simulink library "sm_rollerV_lib_lower_frame_idlerArm_i2u0l3"  (R2026a)
settings: Solver=VariableStepAuto
undefined symbols (not defined in the file): Fixed, Right, Trac
libraries: sm_rollerV_lib_underc_elem x1, sm_rollerV_lib_underc_idlerArm_i2u0l3 x1
Description:
  | Copyright 2024-2026 The MathWorks, Inc.
settings Model: Creator=smiller  LastModifiedBy=smiller

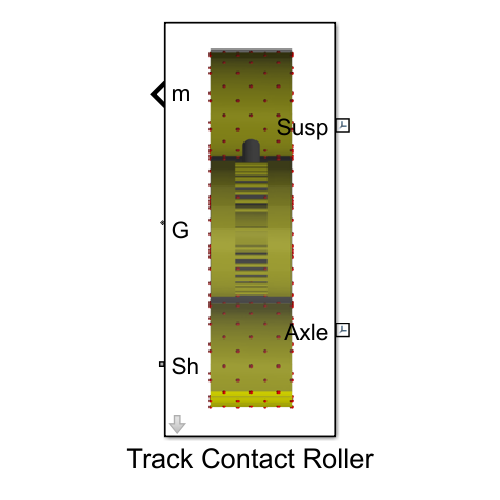
[thumbnail: Simulink's stored preview of the top-level diagram]
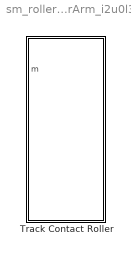
== system sm_rollerV_lib_lower_frame_idlerArm_i2u0l3 ==
  Track Contact Roller : Subsystem  mask(Lower Frame with Roller Point Cloud Contact Geometry){sprk_wid_roll=Trac.Sprocket.Roller.wid, sprk_rad_roll=Trac.Sprocket.Roller.rad, sprk_clr=Trac.Sprocket.Roller.clr, sprk_opc=Trac.Sprocket.Roller.opc, sprk_rad_pitch=Trac.Sprocket.Spoke.pitch_rad, sprk_spoke_rad=Trac.Sprocket.Spoke.rad, sprk_spoke_num=Trac.Sprocket.nSpokes, sprk_spoke_len=Trac.Sprocket.Spoke.len, sprk_rim_spoke_xc=Trac.Sprocket.Rim.spoke_xc, sprk_rim_ir=Trac.Sprocket.Rim.rad_inner, sprk_rim_thk=Trac.Sprocket.Rim.thk, idlerR_rad=Trac.IdlerR.rad, idlerF_rad=Trac.IdlerF.rad, idlerR_total_len=Trac.IdlerR.len_total, idlerF_total_len=Trac.IdlerF.len_total, idlerR_avg_rho=Trac.IdlerR.rho_avg, idlerF_avg_rho=Trac.IdlerF.rho_avg, idlerR_clr=Trac.IdlerR.clr, idlerF_clr=Trac.IdlerF.clr, idlerR_opc=Trac.IdlerR.opc, idlerF_opc=Trac.IdlerF.opc, idlerR_contgeo_ptcld=Trac.IdlerR.ground_contact.ptcld.pts, idlerF_contgeo_ptcld=Trac.IdlerF.ground_contact.ptcld.pts, idlerR_contgeo_rad=Trac.IdlerR.ground_contact.ptcld.rad, idlerF_contgeo_rad=Trac.IdlerF.ground_contact.ptcld.rad, idlerR_contgeo_clr=Trac.IdlerR.belt_contact.clr, idlerF_contgeo_clr=Trac.IdlerF.belt_contact.clr, idlerR_contgeo_opc=Trac.IdlerR.belt_contact.opc, idlerF_contgeo_opc=Trac.IdlerF.belt_contact.opc, arm_idlerc=Trac.IdlerArm.Pivot_to_Idler, arm_tens_x=Trac.IdlerArm.Pivot_to_TensionerX, arm_tens_y=Trac.IdlerArm.Pivot_to_TensionerY, arm_wid=Trac.IdlerArm.wid, arm_thk=Trac.IdlerArm.thk, arm_rho=Trac.IdlerArm.rho, arm_clr=Trac.IdlerArm.clr, arm_opc=Trac.IdlerArm.opc, roller_lower_rad=Trac.Roller.Lower.rad, roller_lower_len=Trac.Roller.Lower.len, roller_lower_rho=Trac.Roller.Lower.rho, roller_lower_clr=Trac.Roller.Lower.clr, roller_lower_opc=Trac.Roller.Lower.opc, roller_lower_contgeo_ptcld=Trac.Roller.Lower.ground_contact.ptcld.pts, roller_lower_contgeo_rad=Trac.Roller.Lower.ground_contact.ptcld.rad, roller_lower_contgeo_clr=Trac.Roller.Lower.belt_contact.clr, roller_lower_contgeo_opc=Trac.Roller.Lower.belt_contact.opc, tensioner_cyl_len=Trac.IdlerF.Tensioner.cyl.len, tensioner_cyl_rad=Trac.IdlerF.Tensioner.cyl.rad, tensioner_cyl_rho=Trac.IdlerF.Tensioner.cyl.rho, tensioner_cyl_clr=Trac.IdlerF.Tensioner.cyl.clr, tensioner_cyl_opc=Trac.IdlerF.Tensioner.cyl.opc, tensioner_pist_len=Trac.IdlerF.Tensioner.piston.len, tensioner_pist_rad=Trac.IdlerF.Tensioner.piston.rad, tensioner_pist_rho=Trac.IdlerF.Tensioner.piston.rho, tensioner_pist_clr=Trac.IdlerF.Tensioner.piston.clr, tensioner_pist_opc=Trac.IdlerF.Tensioner.piston.opc, tensioner_br_len=Trac.IdlerF.Tensioner.bracket.len, tensioner_br_width=Trac.IdlerF.Tensioner.bracket.wid, tensioner_br_height=Trac.IdlerF.Tensioner.bracket.height, tensioner_br_thk=Trac.IdlerF.Tensioner.bracket.thk, tensioner_br_rho=Trac.IdlerF.Tensioner.bracket.rho, tensioner_br_clr=Trac.IdlerF.Tensioner.bracket.clr, tensioner_br_opc=Trac.IdlerF.Tensioner.bracket.opc, tensioner_eqpos=Trac.IdlerF.Tensioner.xeq, tensioner_x0=Trac.IdlerF.Tensioner.x0, tensioner_k=Trac.IdlerF.Tensioner.K, tensioner_b=Trac.IdlerF.Tensioner.B, popup_leftOrRight=Right, popup_trackFrame=Fixed, roller_lower_x=Trac.Frame.SprkOffLon.Lower, idlerFix_x=Trac.Frame.SprkOffLon.IdlerR, idlerArm_x=Trac.Frame.SprkOffLon.IdlerArm, tensionC_x=Trac.Frame.SprkOffLon.TensionC, frame_pivot_x=Trac.Frame.SprkOffLon.PivotFra, axle_x=Trac.Frame.SprkOffLon.Axle, roller_lower_y=Trac.Frame.SprkOffVer.Lower, idlerFix_y=Trac.Frame.SprkOffVer.IdlerR, tensionC_y=Trac.Frame.SprkOffVer.TensionC, frame_pivot_y=Trac.Frame.SprkOffVer.PivotFra, axle_y=Trac.Frame.SprkOffVer.Axle, idlerArm_y=Trac.Frame.SprkOffVer.IdlerArm, frame_mass=Trac.Frame.TrackFrame.Mass, frame_cg_offset=Trac.Frame.TrackFrame.CG, frame_moi=Trac.Frame.TrackFrame.MOI, frame_poi=Trac.Frame.TrackFrame.POI, frame_roller_cg_offset=Trac.Frame.SprkFrame.CG, frame_roller_mass=Trac.Frame.SprkFrame.Mass, frame_roller_moi=Trac.Frame.SprkFrame.MOI, frame_roller_poi=Trac.Frame.SprkFrame.POI, frame_susp_offset=Trac.Frame.SuspOffset, roller_frame_pivot_range=Trac.Frame.PivotFra.Range, roller_frame_pivot_k=Trac.Frame.PivotFra.LimitK, roller_frame_pivot_b=Trac.Frame.PivotFra.LimitB, roller_frame_pivot_tw=Trac.Frame.PivotFra.LimitTW, sprk_rolling_rad=Trac.Sprocket.ground_contact.rolling_radius, roller_lower_rolling_rad=Trac.Roller.Lower.ground_contact.rolling_radius, idlerF_rolling_rad=Trac.IdlerF.ground_contact.rolling_radius, idlerR_rolling_rad=Trac.IdlerR.ground_contact.rolling_radius, rolling_cyl_len=Trac.Belt.w, accent_vis_lext=1e-3, roller_lower_cyl_clr=Trac.Roller.Lower.clr, roller_lower_cyl_opc=Trac.Roller.Lower.opc, idlerR_rollvervis_clr=Trac.IdlerR.clr, idlerF_rollvervis_clr=Trac.IdlerF.clr, idlerR_rollervis_opc=Trac.IdlerR.opc, idlerF_rollervis_opc=Trac.IdlerF.opc, accMn=0.65, accMx=0.75, acc_clr=[0.8 0.8 0.8], acc_opc=1, track_m=Trac.Vis.Track.m, track_cg_offset=Trac.Vis.Track.cg, track_moi=Trac.Vis.Track.moi, track_poi=Trac.Vis.Track.poi, track_xc=Trac.Vis.Track.track_xc, track_clr=Trac.Vis.Track.clr, track_opc=Trac.Vis.Track.opc, popup_sense_roller=Actuator Torque}
      mask prompts: sprk_wid_roll "Roller Width (m)"; sprk_rad_roll "Rolling Radius (m)"; sprk_clr "Color [R G B] (0-1)"; sprk_opc "Opacity (0-1)"; sprk_rad_pitch "Pitch Radius (m)"; sprk_spoke_rad "Radius (m)"; sprk_spoke_num "Number of Spokes"; sprk_spoke_len "Length (m)"; sprk_rim_spoke_xc "Spoke Cross Section [x y] (m)"; sprk_rim_ir "Inner Radius (m)"; sprk_rim_thk "Thickness (m)"; arm_idlerc "Offset Pivot to Idler Center (m)"; arm_tens_x "Offset Pivot to Tensioner Long. (m)"; arm_tens_y "Offset Pivot to Tensioner Vert. (m)"; arm_wid "Idler Arm Width (m)"; arm_thk "Idler Arm Thickness (m)"; arm_rho "Idler Arm Density"; arm_clr "Idler Arm Color [R G B] (m) (0-1)"; arm_opc "Opacity (0-1)"; roller_lower_rad "Radius (m)"; roller_lower_len "Length (m)"; roller_lower_rho "Density (kg/m^3)"; roller_lower_clr "Color [R G B] (0-1)"; roller_lower_opc "Opacity (0-1)"; roller_lower_contgeo_ptcld "Point Cloud [x y z] (m)"; roller_lower_contgeo_rad "Radius (m)"; roller_lower_contgeo_clr "Color [R G B] (0-1)"; roller_lower_contgeo_opc "Opacity (0-1)"; tensioner_cyl_len "Length (m)"; tensioner_cyl_rad "Radius (m)"; tensioner_cyl_rho "Density (kg/m^3)"; tensioner_cyl_clr "Color [R G B] (0-1)"; tensioner_cyl_opc "Opacity (0-1)"; tensioner_pist_len "Piston Length (m)"; tensioner_pist_rad "Radius (m)"; tensioner_pist_rho "Density (kg/m^3)"; tensioner_pist_clr "Color [R G B] (0-1)"; tensioner_pist_opc "Opacity (0.1)"; tensioner_br_len "Length (m)"; tensioner_br_width "Width (m)"; tensioner_br_height "Height (m)"; tensioner_br_thk "Bracket Thickness (m)"; tensioner_br_rho "Density (kg/m^3)"; tensioner_br_clr "Color [R G B] (0-1)"; tensioner_br_opc "Opacity (0.1)"; tensioner_eqpos "Equilibrium Position (m)"; tensioner_x0 "Assembly Position (m)"; tensioner_k "Stiffness Coefficient (N/m)"; tensioner_b "Damping Coefficient (N/(m/s))"; popup_leftOrRight "Left or Right"; popup_trackFrame "Track Frame"; roller_lower_x "Lower Rollers (vector) (m)"; idlerFix_x "Idler Wheel Fixed (m)"; idlerArm_x "Idler Arm (m)"; tensionC_x "Tensioner Cylinder (m)"; frame_pivot_x "Frame Pivot (m)"; axle_x "Axle (m)"; roller_lower_y "Lower Rollers (m)"; idlerFix_y "Idler Wheel Fixed (m)"; tensionC_y "Tensioner Cylinder (m)"; frame_pivot_y "Frame Pivot (m)"; axle_y "Axle (m)"; idlerArm_y "Idler Arm (m)"; frame_mass "Mass (kg)"; frame_cg_offset "CG Offset from Sprocket [x y z] (m)"; frame_moi "Moments of Inertia [Ixx Iyy Izz] (kg*m^2)"; frame_poi "Products of Inertia [Ixx Iyy Izz] (kg*m^2)"; frame_roller_cg_offset "CG Offset from Sprocket [x y z] (m)"; frame_roller_mass "Mass (kg)"; frame_roller_moi "Moments of Inertia [Ixx Iyy Izz] (kg*m^2)"; frame_roller_poi "Products of Inertia [Ixx Iyy Izz] (kg*m^2)"; frame_susp_offset "Suspension Offset from Sprocket [x y z] (m)"; roller_frame_pivot_range "Range (deg)"; roller_frame_pivot_k "Stop stiffness (N*m/deg)"; roller_frame_pivot_b "Stop damping (N*m/(deg*sec)"; roller_frame_pivot_tw "Stop transition width (deg)"; sprk_rolling_rad "Sprocket Rolling Radius (m)"; roller_lower_rolling_rad "Lower Roller Rolling Radius (m)"; idlerF_rolling_rad "Front Idler Rolling Radius (m)"; idlerR_rolling_rad "Rear Idler Rolling Radius (m)"; rolling_cyl_len "Cylinder Length (m)"; accent_vis_lext "Length Extensions (m)"; roller_lower_cyl_clr "Cylinder Color [R G B] (0-1)"; roller_lower_cyl_opc "Cylinder Opacity (0-1)"; accMn "Accent Min Radius (0-1)"; accMx "Accent Max Radius (0-1)"; acc_clr "Accent Color [R G B] (0-1)"; acc_opc "Accent Opacity (0-1)"; track_m "Mass"; track_cg_offset "CG Offset from Sprocket Ctr [x y z] (m)"; track_moi "Moments of Inertia  (kg*m^2)"; track_poi "Products of Inertia  (kg*m^2)"; track_xc "Extrusion Profile [x y] (m)"; track_clr "Color [R G B] (0-1)"; track_opc "Opacity (0-1)"; popup_sense_roller "Roller"
      mask help: Models an undercarriage with rollers that contact the ground via a point cloud. Includes sprocket, rollers, fix idler, and an idler with tensioner. The sprocket has a 1D rotational mechanical interface to the drivetrain.
      mask TypeOptions sprk_wid_roll: Undercarriage/sprk_wid_roll
      mask TypeOptions sprk_rad_roll: Undercarriage/sprk_rad_roll
      mask TypeOptions sprk_clr: Undercarriage/sprk_clr
      mask TypeOptions sprk_opc: Undercarriage/sprk_opc
      mask TypeOptions sprk_rad_pitch: Undercarriage/sprk_rad_pitch
      mask TypeOptions sprk_spoke_rad: Undercarriage/sprk_spoke_rad
      mask TypeOptions sprk_spoke_num: Undercarriage/sprk_spoke_num
      mask TypeOptions sprk_spoke_len: Undercarriage/sprk_spoke_len
      mask TypeOptions sprk_rim_spoke_xc: Undercarriage/sprk_rim_spoke_xc
      mask TypeOptions sprk_rim_ir: Undercarriage/sprk_rim_ir
      mask TypeOptions sprk_rim_thk: Undercarriage/sprk_rim_thk
      mask TypeOptions idlerR_rad: Undercarriage/idlerR_rad
      mask TypeOptions idlerF_rad: Undercarriage/idlerF_rad
      mask TypeOptions idlerR_total_len: Undercarriage/idlerR_total_len
      mask TypeOptions idlerF_total_len: Undercarriage/idlerF_total_len
      mask TypeOptions idlerR_avg_rho: Undercarriage/idlerR_avg_rho
      mask TypeOptions idlerF_avg_rho: Undercarriage/idlerF_avg_rho
      mask TypeOptions idlerR_clr: Undercarriage/idlerR_clr
      mask TypeOptions idlerF_clr: Undercarriage/idlerF_clr
      mask TypeOptions idlerR_opc: Undercarriage/idlerR_opc
      mask TypeOptions idlerF_opc: Undercarriage/idlerF_opc
      mask TypeOptions idlerR_contgeo_ptcld: Undercarriage/idlerR_contgeo_ptcld
      mask TypeOptions idlerF_contgeo_ptcld: Undercarriage/idlerF_contgeo_ptcld
      mask TypeOptions idlerR_contgeo_rad: Undercarriage/idlerR_contgeo_rad
      mask TypeOptions idlerF_contgeo_rad: Undercarriage/idlerF_contgeo_rad
      mask TypeOptions idlerR_contgeo_clr: Undercarriage/idlerR_contgeo_clr
      mask TypeOptions idlerF_contgeo_clr: Undercarriage/idlerF_contgeo_clr
      mask TypeOptions idlerR_contgeo_opc: Undercarriage/idlerR_contgeo_opc
      mask TypeOptions idlerF_contgeo_opc: Undercarriage/idlerF_contgeo_opc
      mask TypeOptions arm_idlerc: Undercarriage/arm_idlerc
      mask TypeOptions arm_tens_x: Undercarriage/arm_tens_x
      mask TypeOptions arm_tens_y: Undercarriage/arm_tens_y
      mask TypeOptions arm_wid: Undercarriage/arm_wid
      mask TypeOptions arm_thk: Undercarriage/arm_thk
      mask TypeOptions arm_rho: Undercarriage/arm_rho
      mask TypeOptions arm_clr: Undercarriage/arm_clr
      mask TypeOptions arm_opc: Undercarriage/arm_opc
      mask TypeOptions roller_lower_rad: Undercarriage/roller_lower_rad
      mask TypeOptions roller_lower_len: Undercarriage/roller_lower_len
      mask TypeOptions roller_lower_rho: Undercarriage/roller_lower_rho
      mask TypeOptions roller_lower_clr: Undercarriage/roller_lower_clr
      mask TypeOptions roller_lower_opc: Undercarriage/roller_lower_opc
      mask TypeOptions roller_lower_contgeo_ptcld: Undercarriage/roller_lower_contgeo_ptcld
      mask TypeOptions roller_lower_contgeo_rad: Undercarriage/roller_lower_contgeo_rad
      mask TypeOptions roller_lower_contgeo_clr: Undercarriage/roller_lower_contgeo_clr
      mask TypeOptions roller_lower_contgeo_opc: Undercarriage/roller_lower_contgeo_opc
      mask TypeOptions tensioner_cyl_len: Undercarriage/tensioner_cyl_len
      mask TypeOptions tensioner_cyl_rad: Undercarriage/tensioner_cyl_rad
      mask TypeOptions tensioner_cyl_rho: Undercarriage/tensioner_cyl_rho
      mask TypeOptions tensioner_cyl_clr: Undercarriage/tensioner_cyl_clr
      mask TypeOptions tensioner_cyl_opc: Undercarriage/tensioner_cyl_opc
      mask TypeOptions tensioner_pist_len: Undercarriage/tensioner_pist_len
      mask TypeOptions tensioner_pist_rad: Undercarriage/tensioner_pist_rad
      mask TypeOptions tensioner_pist_rho: Undercarriage/tensioner_pist_rho
      mask TypeOptions tensioner_pist_clr: Undercarriage/tensioner_pist_clr
      mask TypeOptions tensioner_pist_opc: Undercarriage/tensioner_pist_opc
      mask TypeOptions tensioner_br_len: Undercarriage/tensioner_br_len
      mask TypeOptions tensioner_br_width: Undercarriage/tensioner_br_width
      mask TypeOptions tensioner_br_height: Undercarriage/tensioner_br_height
      mask TypeOptions tensioner_br_thk: Undercarriage/tensioner_br_thk
      mask TypeOptions tensioner_br_rho: Undercarriage/tensioner_br_rho
      mask TypeOptions tensioner_br_clr: Undercarriage/tensioner_br_clr
      mask TypeOptions tensioner_br_opc: Undercarriage/tensioner_br_opc
      mask TypeOptions tensioner_eqpos: Undercarriage/tensioner_eqpos
      mask TypeOptions tensioner_x0: Undercarriage/tensioner_x0
      mask TypeOptions tensioner_k: Undercarriage/tensioner_k
      mask TypeOptions tensioner_b: Undercarriage/tensioner_b
      mask TypeOptions popup_leftOrRight: Undercarriage/popup_leftOrRight
      mask TypeOptions popup_trackFrame: Undercarriage/popup_trackFrame
      mask TypeOptions roller_lower_x: Undercarriage/roller_lower_x
      mask TypeOptions idlerFix_x: Undercarriage/idlerFix_x
      mask TypeOptions idlerArm_x: Undercarriage/idlerArm_x
      mask TypeOptions tensionC_x: Undercarriage/tensionC_x
      mask TypeOptions frame_pivot_x: Undercarriage/frame_pivot_x
      mask TypeOptions axle_x: Undercarriage/axle_x
      mask TypeOptions roller_lower_y: Undercarriage/roller_lower_y
      mask TypeOptions idlerFix_y: Undercarriage/idlerFix_y
      mask TypeOptions tensionC_y: Undercarriage/tensionC_y
      mask TypeOptions frame_pivot_y: Undercarriage/frame_pivot_y
      mask TypeOptions axle_y: Undercarriage/axle_y
      mask TypeOptions idlerArm_y: Undercarriage/idlerArm_y
      mask TypeOptions frame_mass: Undercarriage/frame_mass
      mask TypeOptions frame_cg_offset: Undercarriage/frame_cg_offset
      mask TypeOptions frame_moi: Undercarriage/frame_moi
      mask TypeOptions frame_poi: Undercarriage/frame_poi
      mask TypeOptions frame_roller_cg_offset: Undercarriage/frame_roller_cg_offset
      mask TypeOptions frame_roller_mass: Undercarriage/frame_roller_mass
      mask TypeOptions frame_roller_moi: Undercarriage/frame_roller_moi
      mask TypeOptions frame_roller_poi: Undercarriage/frame_roller_poi
      mask TypeOptions frame_susp_offset: Undercarriage/frame_susp_offset
      mask TypeOptions roller_frame_pivot_range: Undercarriage/roller_frame_pivot_range
      mask TypeOptions roller_frame_pivot_k: Undercarriage/roller_frame_pivot_k
      mask TypeOptions roller_frame_pivot_b: Undercarriage/roller_frame_pivot_b
      mask TypeOptions roller_frame_pivot_tw: Undercarriage/roller_frame_pivot_tw
      mask TypeOptions sprk_rolling_rad: Undercarriage/sprk_rolling_rad
      mask TypeOptions roller_lower_rolling_rad: Undercarriage/roller_lower_rolling_rad
      mask TypeOptions idlerF_rolling_rad: Undercarriage/idlerF_rolling_rad
      mask TypeOptions idlerR_rolling_rad: Undercarriage/idlerR_rolling_rad
      mask TypeOptions rolling_cyl_len: Undercarriage/rolling_cyl_len
      mask TypeOptions accent_vis_lext: Undercarriage/accent_vis_lext
      mask TypeOptions roller_lower_cyl_clr: Undercarriage/roller_lower_cyl_clr
      mask TypeOptions roller_lower_cyl_opc: Undercarriage/roller_lower_cyl_opc
      mask TypeOptions idlerR_rollvervis_clr: Undercarriage/idlerR_rollvervis_clr
      mask TypeOptions idlerF_rollvervis_clr: Undercarriage/idlerF_rollvervis_clr
      mask TypeOptions idlerR_rollervis_opc: Undercarriage/idlerR_rollervis_opc
      mask TypeOptions idlerF_rollervis_opc: Undercarriage/idlerF_rollervis_opc
      mask TypeOptions accMn: Undercarriage/accMn
      mask TypeOptions accMx: Undercarriage/accMx
      mask TypeOptions acc_clr: Undercarriage/acc_clr
      mask TypeOptions acc_opc: Undercarriage/acc_opc
      mask TypeOptions track_m: Track/track_m
      mask TypeOptions track_cg_offset: Track/track_cg_offset
      mask TypeOptions track_moi: Track/track_moi
      mask TypeOptions track_poi: Track/track_poi
      mask TypeOptions track_xc: Track/track_xc
      mask TypeOptions track_clr: Track/track_clr
      mask TypeOptions track_opc: Track/track_opc
      mask TypeOptions popup_sense_roller: Undercarriage/popup_sense_roller
      mask DialogControl cont_sprocket Prompt: Sprocket
      mask DialogControl cont_sprk_roller Prompt: Roller
      mask DialogControl cont_sprk_spoke Prompt: Spoke
      mask DialogControl cont_sprk_rim Prompt: Rim
      mask DialogControl cont_idler Prompt: Idler
      mask DialogControl cont_idler_roller Prompt: Roller
      mask DialogControl text_idler_rear Prompt: Rear
      mask DialogControl text_idler_front Prompt: Front
      mask DialogControl text_idler_rad Prompt: Radius (m)
      mask DialogControl text_idler_len Prompt: Total Length (m)
      mask DialogControl text_idler_rho_avg Prompt: Avg Density (kg/m^3)
      mask DialogControl text_idler_wheel_clr_copy Prompt: Color [R G B] (0-1)
      mask DialogControl text_idler_opc Prompt: Opacity (0-1)
      mask DialogControl cont_idler_pin_contgeo Prompt: Contact Geometry
      mask DialogControl text_idler_contgeo_ptcld Prompt: Point Cloud [x y z] (m)
      mask DialogControl text_idler_contgeo_rad Prompt: Radius (m)
      mask DialogControl text_idler_contgeo_clr Prompt: Color [R G B] (0-1)
      mask DialogControl text_idler_contgeo_opc Prompt: Opacity (0-1)
      mask DialogControl cont_idler_arm Prompt: Idler Arm
      mask DialogControl cont_roller_lower Prompt: Rollers
      mask DialogControl cont_rollerL_roller Prompt: Lower
      mask DialogControl cont_rollerL_contgeo Prompt: Contact Geometry
      mask DialogControl cont_tensioner Prompt: Tensioner
      mask DialogControl cont_tens_cyl Prompt: Cylinder
      mask DialogControl cont_tens_pist Prompt: Piston
      mask DialogControl cont_tens_brk Prompt: Bracket
      mask DialogControl cont_tens_asy Prompt: Assembly
      mask DialogControl cont_frame Prompt: Frame
      mask DialogControl cont_frame_lon Prompt: Longitudinal Offsets from Sprocket
      mask DialogControl cont_frame_ver Prompt: Vertical Offsets from Sprocket
      mask DialogControl cont_frame_mass Prompt: Mass and Inertia
      mask DialogControl cont_sprocket_frame Prompt: Sprocket Frame
      mask DialogControl cont_roller_frame Prompt: Roller Frame
      mask DialogControl cont_susp_offset Prompt: Suspension Offsets
      mask DialogControl cont_frame_pivot Prompt: Frame Pivot
      mask DialogControl cont_rolling Prompt: Rolling
      mask DialogControl cont_constraints_length Prompt: Constraints and Length
      mask DialogControl cont_rollervis_roller Prompt: Roller Visual: Roller
      mask DialogControl cont_rollervis_idler Prompt: Roller Visual: Idler
      mask DialogControl text_rollervis_idler_rear Prompt: Rear
      mask DialogControl text_rollervis_idler_front Prompt: Front
      mask DialogControl text_rollervis_idler_clr Prompt: Color [R G B] (0-1)
      mask DialogControl text_rollervis_idler_opc Prompt: Opacity (0-1)
      mask DialogControl cont_accentvis Prompt: Accent Visual
      mask DialogControl cont_belt Prompt: Belt
      mask DialogControl cont_sensing Prompt: Sensing
      mask Display: image('sm_roller_ptcld_lowerframe_idlerarm_i2u0l3_IMAGE.png')

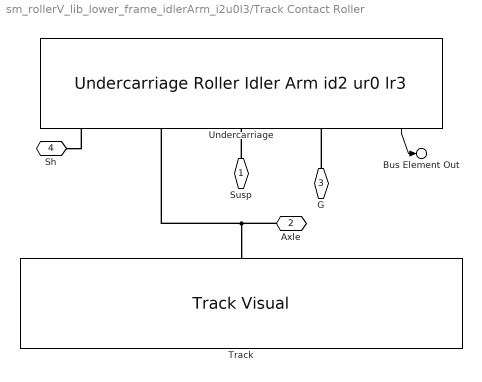
== system sm_rollerV_lib_lower_frame_idlerArm_i2u0l3/Track Contact Roller ==
  Track : sm_rollerV_lib_underc_elem/Track Visual  track_m=track_m  track_cg_offset=track_cg_offset  track_axle_offset_x=Trac.Frame.SprkOffLon.Axle  track_axle_offset_y=Trac.Frame.SprkOffVer.Axle  track_moi=track_moi  track_poi=track_poi  track_xc=track_xc  track_w=Trac.Belt.w  track_clr=track_clr  track_opc=track_opc
  Undercarriage : sm_rollerV_lib_underc_idlerArm_i2u0l3/Undercarriage Roller Idler Arm id2 ur0 lr3  popup_leftOrRight=Right  sprk_rad_roll=sprk_rad_roll  sprk_wid_roll=sprk_wid_roll  sprk_clr=sprk_clr  sprk_opc=sprk_opc  sprk_rim_ir=sprk_rim_ir  sprk_rim_thk=sprk_rim_thk  sprk_rim_spoke_xc=sprk_rim_spoke_xc  sprk_rad_pitch=sprk_rad_pitch  sprk_spoke_rad=sprk_spoke_rad  sprk_spoke_len=sprk_spoke_len  sprk_spoke_num=sprk_spoke_num  idlerR_rad=idlerR_rad  idlerF_rad=idlerF_rad  idlerR_total_len=idlerR_total_len  idlerF_total_len=idlerF_total_len  idlerR_avg_rho=idlerR_avg_rho  idlerF_avg_rho=idlerF_avg_rho  idlerR_clr=idlerR_clr  idlerF_clr=idlerF_clr  idlerR_opc=idlerR_opc  idlerF_opc=idlerF_opc  idlerR_contgeo_ptcld=idlerR_contgeo_ptcld  idlerF_contgeo_ptcld=idlerF_contgeo_ptcld  idlerR_contgeo_rad=idlerR_contgeo_rad  idlerF_contgeo_rad=idlerF_contgeo_rad  idlerR_contgeo_clr=idlerR_contgeo_clr  idlerF_contgeo_clr=idlerF_contgeo_clr  idlerR_contgeo_opc=idlerR_contgeo_opc  idlerF_contgeo_opc=idlerF_contgeo_opc  arm_idlerc=arm_idlerc  arm_tens_x=arm_tens_x  arm_tens_y=arm_tens_y  arm_wid=arm_wid  arm_thk=arm_thk  arm_rho=arm_rho  arm_clr=arm_clr  arm_opc=arm_opc  roller_lower_len=roller_lower_len  roller_lower_rad=roller_lower_rad  roller_lower_rho=roller_lower_rho  roller_lower_clr=roller_lower_clr  roller_lower_opc=roller_lower_opc  roller_lower_contgeo_clr=roller_lower_contgeo_clr  roller_lower_contgeo_opc=roller_lower_contgeo_opc  roller_lower_contgeo_ptcld=roller_lower_contgeo_ptcld  roller_lower_contgeo_rad=roller_lower_contgeo_rad  tensioner_cyl_len=tensioner_cyl_len  tensioner_cyl_rad=tensioner_cyl_rad  tensioner_cyl_rho=tensioner_cyl_rho  tensioner_cyl_clr=tensioner_cyl_clr  tensioner_cyl_opc=tensioner_cyl_opc  tensioner_pist_len=tensioner_pist_len  tensioner_pist_rad=tensioner_pist_rad  tensioner_pist_rho=tensioner_pist_rho  tensioner_pist_clr=tensioner_pist_clr  tensioner_pist_opc=tensioner_pist_opc  tensioner_br_len=tensioner_br_len  tensioner_br_width=tensioner_br_width  tensioner_br_height=tensioner_br_height  tensioner_br_thk=tensioner_br_thk  tensioner_br_rho=tensioner_br_rho  tensioner_br_clr=tensioner_br_clr  tensioner_br_opc=tensioner_br_opc  tensioner_eqpos=tensioner_eqpos  tensioner_x0=tensioner_x0  tensioner_k=tensioner_k  tensioner_b=tensioner_b  popup_trackFrame=Fixed  roller_lower_x=roller_lower_x  axle_x=axle_x  idlerFix_x=idlerFix_x  frame_pivot_x=frame_pivot_x  tensionC_x=tensionC_x  idlerArm_x=idlerArm_x  roller_lower_y=roller_lower_y  axle_y=axle_y  idlerArm_y=idlerArm_y  idlerFix_y=idlerFix_y  frame_pivot_y=frame_pivot_y  tensionC_y=tensionC_y  frame_cg_offset=frame_cg_offset  frame_mass=frame_mass  frame_moi=frame_moi  frame_poi=frame_poi  frame_roller_cg_offset=frame_roller_cg_offset  frame_roller_mass=frame_roller_mass  frame_roller_moi=frame_roller_moi  frame_roller_poi=frame_roller_poi  frame_susp_offset=frame_susp_offset  roller_frame_pivot_range=roller_frame_pivot_range  roller_frame_pivot_k=roller_frame_pivot_k  roller_frame_pivot_b=roller_frame_pivot_b  roller_frame_pivot_tw=roller_frame_pivot_tw  sprk_rolling_rad=sprk_rolling_rad  roller_lower_rolling_rad=roller_lower_rolling_rad  idlerF_rolling_rad=idlerF_rolling_rad  idlerR_rolling_rad=idlerR_rolling_rad  rolling_cyl_len=rolling_cyl_len  accent_vis_lext=accent_vis_lext  roller_lower_cyl_clr=roller_lower_cyl_clr  roller_lower_cyl_opc=roller_lower_cyl_opc  idlerR_rollvervis_clr=idlerR_rollvervis_clr  idlerF_rollvervis_clr=idlerF_rollvervis_clr  idlerR_rollervis_opc=idlerR_rollervis_opc  idlerF_rollervis_opc=idlerF_rollervis_opc  accMn=accMn  accMx=accMx  acc_clr=acc_clr  acc_opc=acc_opc  popup_sense_roller=Actuator Torque
  Susp : PMIOPort  Side=Left
  Axle : PMIOPort  Port=2  Side=Left
  G : PMIOPort  Port=3  Side=Right
  Sh : PMIOPort  Port=4  Side=Right
  Bus Element Out : Outport  PortName=m  Element=Underc
  wires:
  Undercarriage/1 -> Bus Element Out/1
  connections:
  Axle/RConn1 -- Undercarriage/RConn3 -- Track/LConn1
  Sh/RConn1 -- Undercarriage/RConn4
  Susp/RConn1 -- Undercarriage/RConn2
  G/RConn1 -- Undercarriage/RConn1
